simulink model "display_data"  (R2024a)
settings: Solver=VariableStepAuto  StartTime=0.0  StopTime=inf  RelTol=1e-3
libraries: ros2lib x5
settings Model: Creator=eswarm  LastModifiedBy=eswarm

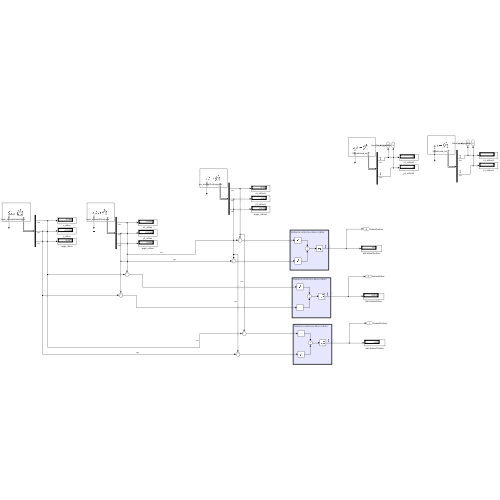
[thumbnail: Simulink's stored preview of the top-level diagram]
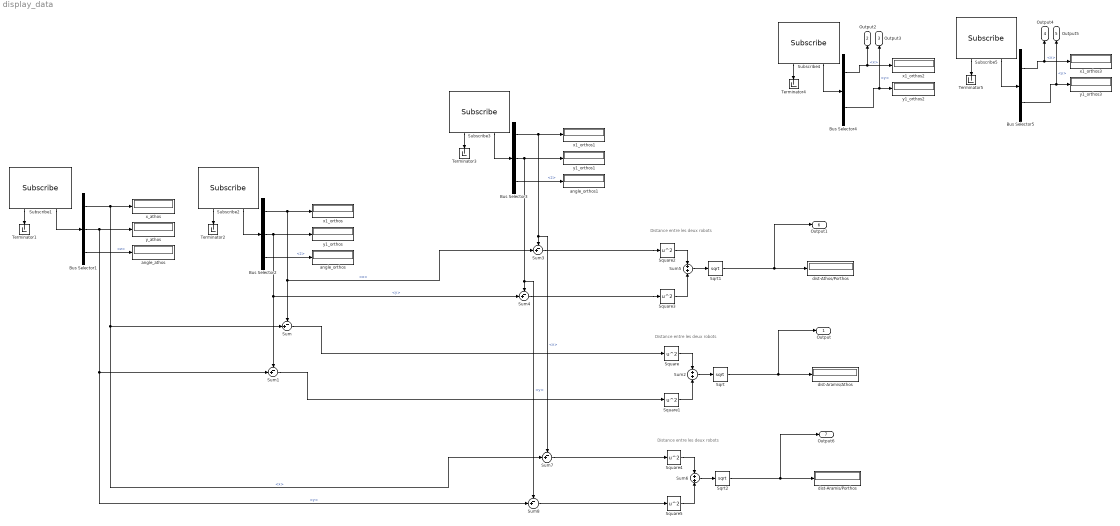
== system display_data ==
  note: Distance entre les deux robots
  note: Distance entre les deux robots
  note: Distance entre les deux robots
  Bus Selector1 : BusSelector  OutputSignals=pose.position.x,pose.position.y,pose.orientation.z
  Bus Selector2 : BusSelector  OutputSignals=pose.position.x,pose.position.y,pose.orientation.z
  Bus Selector3 : BusSelector  OutputSignals=pose.position.x,pose.position.y,pose.orientation.z
  Bus Selector4 : BusSelector  OutputSignals=linear.x,linear.y
  Bus Selector5 : BusSelector  OutputSignals=linear.x,linear.y
  Sqrt : Sqrt
  Sqrt1 : Sqrt
  Sqrt2 : Sqrt
  Square{,1..5} (6 alike) : Math  Operator=square
  Subscribe1 : ros2lib/Subscribe  topicSource=Select from ROS network  topic=/vrpn_mocap/Aramis/pose  messageType=geometry_msgs/PoseStamped  sampleTime=0.1  QOSHistory=Keep last  QOSDepth=1  QOSReliability=Best effort  QOSDurability=Volatile  QOSDeadline=Inf  QOSLifespan=Inf  QOSLiveliness=Automatic  QOSLeaseDuration=Inf  QOSAvoidROSNamespaceConventions=off
  Subscribe2 : ros2lib/Subscribe  topicSource=Select from ROS network  topic=/vrpn_mocap/Athos/pose  messageType=geometry_msgs/PoseStamped  sampleTime=0.1  QOSHistory=Keep last  QOSDepth=1  QOSReliability=Best effort  QOSDurability=Volatile  QOSDeadline=Inf  QOSLifespan=Inf  QOSLiveliness=Automatic  QOSLeaseDuration=Inf  QOSAvoidROSNamespaceConventions=off
  Subscribe3 : ros2lib/Subscribe  topicSource=Select from ROS network  topic=/vrpn_mocap/Porthos/pose  messageType=geometry_msgs/PoseStamped  sampleTime=0.1  QOSHistory=Keep last  QOSDepth=1  QOSReliability=Best effort  QOSDurability=Volatile  QOSDeadline=Inf  QOSLifespan=Inf  QOSLiveliness=Automatic  QOSLeaseDuration=Inf  QOSAvoidROSNamespaceConventions=off
  Subscribe4 : ros2lib/Subscribe  topicSource=Select from ROS network  topic=/Aramis/cmd_vel  messageType=geometry_msgs/Twist  sampleTime=0.1  QOSHistory=Keep last  QOSDepth=1  QOSReliability=Best effort  QOSDurability=Volatile  QOSDeadline=Inf  QOSLifespan=Inf  QOSLiveliness=Automatic  QOSLeaseDuration=Inf  QOSAvoidROSNamespaceConventions=off
  Subscribe5 : ros2lib/Subscribe  topicSource=Select from ROS network  topic=/Athos/cmd_vel  messageType=geometry_msgs/Twist  sampleTime=0.1  QOSHistory=Keep last  QOSDepth=1  QOSReliability=Best effort  QOSDurability=Volatile  QOSDeadline=Inf  QOSLifespan=Inf  QOSLiveliness=Automatic  QOSLeaseDuration=Inf  QOSAvoidROSNamespaceConventions=off
  Sum{,1,3..4,7..8} (6 alike) : Sum  Inputs=-+|
  Sum2 : Sum  Inputs=+|+
  Sum5 : Sum  Inputs=+|+
  Sum6 : Sum  Inputs=+|+
  Terminator{1..5} (5 alike) : Terminator
  angle_athos : Display
  angle_orthos : Display
  angle_orthos1 : Display
  dist-Aramis/Athos : Display
  dist-Aramis/Porthos : Display
  dist-Athos/Porthos : Display
  x1_orthos{,1..3} (4 alike) : Display
  x_athos : Display
  y1_orthos{,1..3} (4 alike) : Display
  y_athos : Display
  Output : Outport  SignalName=Aramis/Athos
  Output2 : Outport  Port=2  SignalName=linear_x_aramis
  Output3 : Outport  Port=3  SignalName=linear_y_aramis
  Output4 : Outport  Port=4  SignalName=linear_x_athos
  Output5 : Outport  Port=5  SignalName=linear_y_athos
  Output1 : Outport  Port=6  SignalName=Athos/Porthos
  Output6 : Outport  Port=7  SignalName=Aramis/Porthos
  wires:
  Sum1/1 -> Square1/1
  Bus Selector5/2 -> Output5/1, y1_orthos3/1  "<y>"
  Subscribe5/1 -> Terminator5/1
  Subscribe1/1 -> Terminator1/1
  Subscribe2/2 -> Bus Selector2/1
  Bus Selector5/1 -> Output4/1, x1_orthos3/1  "<x>"
  Bus Selector1/3 -> angle_athos/1  "<z>"
  Bus Selector2/3 -> angle_orthos/1  "<z>"
  Square1/1 -> Sum2/2
  Subscribe5/2 -> Bus Selector5/1
  Bus Selector4/2 -> Output3/1, y1_orthos2/1  "<y>"
  Subscribe1/2 -> Bus Selector1/1
  Sum2/1 -> Sqrt/1
  Subscribe4/1 -> Terminator4/1
  Bus Selector4/1 -> Output2/1, x1_orthos2/1  "<x>"
  Sum/1 -> Square/1
  Square/1 -> Sum2/1
  Subscribe2/1 -> Terminator2/1
  Sqrt/1 -> Output/1, dist-Aramis/Athos/1
  Subscribe4/2 -> Bus Selector4/1
  Subscribe3/1 -> Terminator3/1
  Subscribe3/2 -> Bus Selector3/1
  Bus Selector2/1 -> Sum3/2, Sum/1, x1_orthos/1  "<x>"
  Bus Selector3/3 -> angle_orthos1/1  "<z>"
  Bus Selector2/2 -> Sum4/2, Sum1/1, y1_orthos/1  "<y>"
  Sum5/1 -> Sqrt1/1
  Sum4/1 -> Square3/1
  Sum3/1 -> Square2/1
  Sqrt1/1 -> Output1/1, dist-Athos/Porthos/1
  Square2/1 -> Sum5/1
  Square3/1 -> Sum5/2
  Sum6/1 -> Sqrt2/1
  Sqrt2/1 -> Output6/1, dist-Aramis/Porthos/1
  Square4/1 -> Sum6/1
  Square5/1 -> Sum6/2
  Sum8/1 -> Square5/1
  Bus Selector3/2 -> Sum8/1, Sum4/1, y1_orthos1/1  "<y>"
  Bus Selector3/1 -> Sum7/1, Sum3/1, x1_orthos1/1  "<x>"
  Bus Selector1/2 -> Sum8/2, Sum1/2, y_athos/1  "<y>"
  Bus Selector1/1 -> Sum7/2, Sum/2, x_athos/1  "<x>"
  Sum7/1 -> Square4/1
